simulink model "Sem2_Task1"  (R2017b)
settings: Solver=VariableStepAuto  StartTime=0.0  StopTime=30.0  RelTol=1e-3
libraries: simulink x4
settings Model: Creator=fedor  LastModifiedBy=fedor

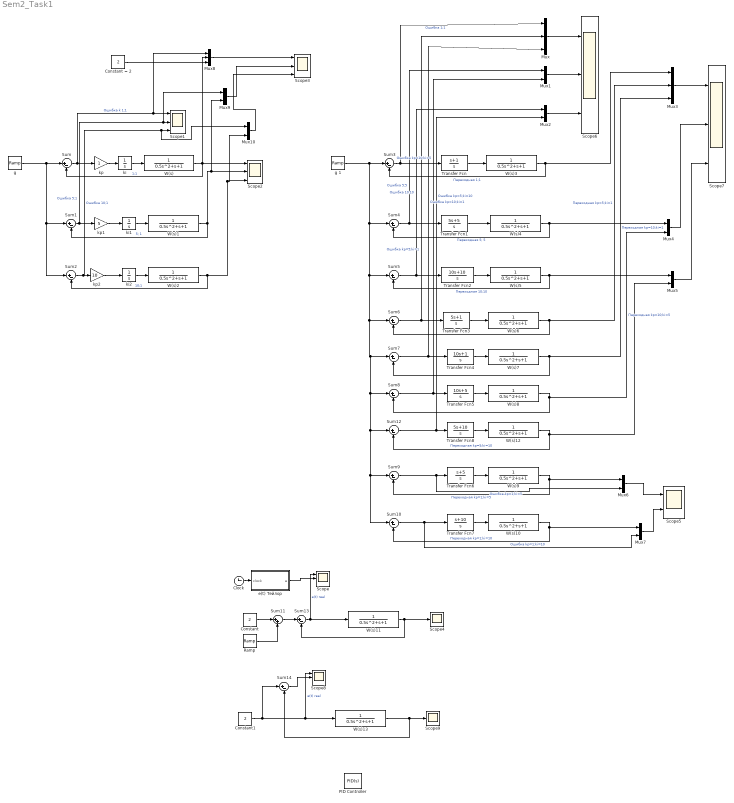
== system Sem2_Task1 ==
  Clock : Clock
  Constant : Constant  Value=2
  Constant = 2 : Constant  Value=2
  Constant1 : Constant  Value=2
  Mux : Mux  Inputs=3
  Mux{1..2,4..7,9..10} (8 alike) : Mux  Inputs=2
  Mux3 : Mux  Inputs=3
  Mux8 : Mux  Inputs=3
  PID Controller : simulink/Continuous/PID Controller  Controller=PID  TimeDomain=Continuous-time  SampleTime=-1  IntegratorMethod=Forward Euler  FilterMethod=Forward Euler  Form=Parallel  UseFilter=on  ControllerParametersSource=internal  P=1  I=1  D=0  N=100  InitialConditionSource=internal  InitialConditionForIntegrator=0  InitialConditionForFilter=0  ExternalReset=none  LimitOutput=off  UpperSaturationLimit=inf  LowerSaturationLimit=-inf  LinearizeAsGain=on  AntiWindupMode=none  Kb=1  TrackingMode=off  Kt=1  PParamMin=[]  PParamMax=[]  IParamMin=[]  IParamMax=[]  DParamMin=[]  DParamMax=[]  NParamMin=[]  NParamMax=[]  KbParamMin=[]  KbParamMax=[]  KtParamMin=[]  KtParamMax=[]  POutMin=[]  POutMax=[]  IOutMin=[]  IOutMax=[]  DOutMin=[]  DOutMax=[]  NOutMin=[]  NOutMax=[]  KbOutMin=[]  KbOutMax=[]  KtOutMin=[]  KtOutMax=[]  IntegratorOutMin=[]  IntegratorOutMax=[]  FilterOutMin=[]  FilterOutMax=[]  SumOutMin=[]  SumOutMax=[]  SumI1OutMin=[]  SumI1OutMax=[]  SumI2OutMin=[]  SumI2OutMax=[]  SumI3OutMin=[]  SumI3OutMax=[]  SumDOutMin=[]  SumDOutMax=[]  SaturationOutMin=[]  SaturationOutMax=[]  IntegratorContinuousStateAttributes=''  IntegratorStateMustResolveToSignalObject=off  IntegratorRTWStateStorageClass=Auto  FilterContinuousStateAttributes=''  FilterStateMustResolveToSignalObject=off  FilterRTWStateStorageClass=Auto  DifferentiatorICPrevScaledInput=0  DifferentiatorOutMin=[]  DifferentiatorOutMax=[]  InitialConditionSetting=State (most efficient)  FilterDiffOutCoefMin=[]  FilterDiffOutCoefMax=[]  SumDenOutMin=[]  SumDenOutMax=[]  SumNumOutMin=[]  SumNumOutMax=[]  ReciprocalOutMin=[]  ReciprocalOutMax=[]  DivideOutMin=[]  DivideOutMax=[]  TunerSelectOption=Transfer Function Based (PID Tuner App)
  Ramp : simulink/Sources/Ramp  slope=0.3  start=0  X0=0
  Scope{,1..3,6..8} (7 alike) : Scope  NumInputPorts=3
  Scope4 : Scope
  Scope5 : Scope  NumInputPorts=2
  Scope9 : Scope
  Sum{,1..10,12..14} (14 alike) : Sum  Inputs=|+-
  Sum11 : Sum  Inputs=|++
  Transfer Fcn : TransferFcn  Numerator=[1 1]  Denominator=[1 0]
  Transfer Fcn1 : TransferFcn  Numerator=[5 5]  Denominator=[1 0]
  Transfer Fcn2 : TransferFcn  Numerator=[10 10]  Denominator=[1 0]
  Transfer Fcn3 : TransferFcn  Numerator=[5 1]  Denominator=[1 0]
  Transfer Fcn4 : TransferFcn  Numerator=[10 1]  Denominator=[1 0]
  Transfer Fcn5 : TransferFcn  Numerator=[10 5]  Denominator=[1 0]
  Transfer Fcn6 : TransferFcn  Numerator=[1 5]  Denominator=[1 0]
  Transfer Fcn7 : TransferFcn  Numerator=[1 10]  Denominator=[1 0]
  Transfer Fcn8 : TransferFcn  Numerator=[5 10]  Denominator=[1 0]
  W(s){,1..13} (14 alike) : TransferFcn  Denominator=[0.5 1 1]
  e(t) Тейлор : MATLAB Function  TreatAsAtomicUnit=on
  "g " : simulink/Sources/Ramp  slope=2  start=0  X0=0
  g 1 : simulink/Sources/Ramp  slope=2  start=0  X0=0
  ki : Integrator
  ki1 : Integrator
  ki2 : Integrator
  kp : Gain
  kp1 : Gain  Gain=5
  kp2 : Gain  Gain=10
  wires:
  kp/1 -> ki/1
  ki/1 -> W(s)/1
  W(s)/1 -> Mux8/2, Scope2/1, Sum/2  "1;1"
  "g "/1 -> Sum2/1, Sum1/1, Sum/1
  W(s)1/1 -> Mux9/2, Scope2/2, Sum1/2  "5; 1"
  Sum1/1 -> Mux9/1, Scope1/2, kp1/1  "Ошибка 5;1"
  ki1/1 -> W(s)1/1
  kp1/1 -> ki1/1
  kp2/1 -> ki2/1
  ki2/1 -> W(s)2/1
  Sum2/1 -> Mux10/1, Scope1/3, kp2/1  "Ошибка 10;1"
  W(s)2/1 -> Mux10/2, Scope2/3, Sum2/2  "10;1"
  Sum/1 -> Mux8/1, Scope1/1, kp/1  "Ошибка k 1;1"
  Sum3/1 -> Mux/1, Transfer Fcn/1  "Ошибка 1;1"
  W(s)5/1 -> Mux5/1, Sum5/2  "Переходная 10;10"
  Sum5/1 -> Mux2/1, Transfer Fcn2/1  "Ошибка 10;10"
  Sum4/1 -> Mux1/1, Transfer Fcn1/1  "Ошибка 5;5"
  W(s)4/1 -> Sum4/2, Mux4/1  "Переходная 5; 5"
  W(s)3/1 -> Sum3/2, Mux3/1  "Переходная 1;1"
  Transfer Fcn/1 -> W(s)3/1
  Transfer Fcn1/1 -> W(s)4/1
  Transfer Fcn2/1 -> W(s)5/1
  Transfer Fcn3/1 -> W(s)6/1
  W(s)6/1 -> Mux3/2, Sum6/2  "Переходная kp=5;ki=1"
  Sum6/1 -> Mux/2, Transfer Fcn3/1  "Ошибка kp=5;ki=1"
  W(s)7/1 -> Mux3/3, Sum7/2  "Переходная kp=10;ki=1"
  Transfer Fcn4/1 -> W(s)7/1
  Sum7/1 -> Mux/3, Transfer Fcn4/1  "Ошибка kp=10;ki=1"
  Sum8/1 -> Mux1/2, Transfer Fcn5/1  "Ошибка kp=10;ki=5"
  Transfer Fcn5/1 -> W(s)8/1
  W(s)8/1 -> Mux4/2, Sum8/2  "Переходная kp=10;ki=5"
  W(s)9/1 -> Mux6/1, Sum9/2  "Переходная kp=1;ki=5"
  Transfer Fcn6/1 -> W(s)9/1
  Sum9/1 -> Mux6/2, Transfer Fcn6/1  "Ошибка kp=1;ki=5"
  Sum10/1 -> Mux7/2, Transfer Fcn7/1  "Ошибка kp=1;ki=10"
  Transfer Fcn7/1 -> W(s)10/1
  W(s)10/1 -> Mux7/1, Sum10/2  "Переходная kp=1;ki=10"
  g 1/1 -> Sum3/1, Sum4/1, Sum10/1, Sum9/1, Sum12/1, Sum8/1, Sum7/1, Sum6/1, Sum5/1
  Sum12/1 -> Mux2/2, Transfer Fcn8/1  "Ошибка kp=5;ki=10"
  Transfer Fcn8/1 -> W(s)12/1
  W(s)12/1 -> Mux5/2, Sum12/2  "Переходная kp=5;ki=10"
  Mux1/1 -> Scope6/2
  Mux/1 -> Scope6/1
  Mux2/1 -> Scope6/3
  Mux5/1 -> Scope7/3
  Mux3/1 -> Scope7/1
  Mux4/1 -> Scope7/2
  Mux6/1 -> Scope5/1
  Mux7/1 -> Scope5/2
  Mux8/1 -> Scope3/1
  Mux9/1 -> Scope3/2
  Mux10/1 -> Scope3/3
  Constant = 2/1 -> Mux8/3
  Constant/1 -> Sum11/1
  Ramp/1 -> Sum11/2
  Sum11/1 -> Sum13/1
  W(s)11/1 -> Sum13/2, Scope4/1
  Clock/1 -> e(t) Тейлор/1(clock)
  e(t) Тейлор/1(e) -> Scope/2
  Sum13/1 -> W(s)11/1, Scope/1  "e(t) real"
  Constant1/1 -> Sum14/1, Scope8/1, W(s)13/1  "e(t) real"
  W(s)13/1 -> Sum14/2, Scope9/1
  Sum14/1 -> Scope8/2

== matlab function Sem2_Task1/e(t) Тейлор ==
  data: clock input; e output
function e  = fcn(clock)
e =(3+2*(20+3*clock))/40;
